simulink model "Model_120S2P"  (R2019b)
settings: Solver=VariableStepAuto  StartTime=0.0  StopTime=800  RelTol=1e-3
libraries: fl_lib x29, nesl_utility x6, simulink x2, hwlogiciolib x1, ee_lib x1
(part 3 of 3)

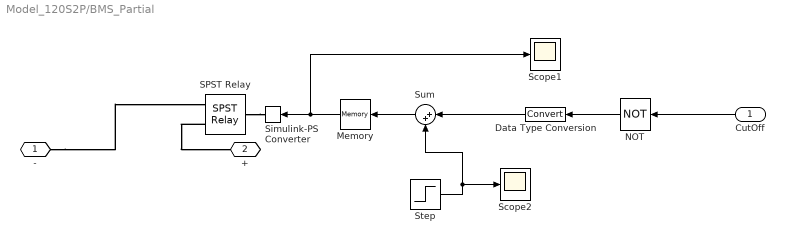
== system Model_120S2P/BMS_Partial ==
  CutOff : Inport
  Data Type Conversion : DataTypeConversion
  Memory : Memory  InheritSampleTime=on  LinearizeMemory=on  LinearizeAsDelay=on
  NOT : Logic  Operator=NOT  IconShape=distinctive  AllPortsSameDT=off  OutDataTypeStr=boolean
  SPST Relay : ee_lib/Switches & Breakers/Relays/SPST Relay  block_choices=ee.enum.controlport.ps  R_closed=0.01 Ohm  G_open=1e-8 1/Ohm  Threshold=0.5  exposemeasurement=ee.enum.exposemeasurement.hidden  T_brk_C_S=0 s  T_mak_C_S=0 s  V_rated=5 V  V_energize=75  V_deenergize=25  l_winding=0.08 H  r_winding=12.5 Ohm  g_winding=1e-9 1/Ohm  enable_faults=ee.enum.relays.enable.no  fault_action=ee.enum.relays.faultaction.none  fault_types=ee.enum.relays.faultTypes.winding  fault_condition_ps=ee.enum.relays.faultConditionSPSTps.csstuck  r_deg_closed_s=1e-9 Ohm  winding_tau_fault=1e-3 s  tau_fault=1e-3 s  enable_temporal_fault=ee.enum.relays.enable.no  t_fault_stick=1 s  t_fault_ComOpen=1 s  t_fault=1 s  enable_behavioral_fault=ee.enum.relays.enable.no  winding_max_permissible_voltage=inf V  n_fail_on_voltage=1  winding_max_permissible_current=inf A  max_permissible_current=inf A  t_fail_on_current=1 s
      settings: SourceProductName=Simscape Electrical  SourceProductBaseCode=PS  InternalSimscapePortConfiguration="{\"Bottom\":[],\"Left\":[{\"id\":\"PS\",\"label\":\"PS\",\"type\":\"input\"}],\"Right\":[{\"id\":\"S\",\"label\":\"S\",\"type\":\"foundation.electrical.electrical\"},{\"id\":\"COM\",\"label\":\"C\",\"type\":\"foundation.electrical.electrical\"}],\"Top\":[]}"
  Scope1 : Scope
  Scope2 : Scope
  Simulink-PS Converter : nesl_utility/Simulink-PS Converter  PhysicalDomain=network_engine_domain  SubClassName=ps_input  LeftPortType=input  RightPortType=output  PseudoPeriodic=off  Frequencies=[]  NoiseDistribution=none  NoiseParameters=[]  Unit=1  AffineConversion=off  FilteringAndDerivatives=provide  SimscapeFilterOrder=1  InputFilterTimeConstant=0.001  UdotUserProvided=0
  Step : Step  Time=10  Before=1  After=0  SampleTime=0
  Sum : Sum  Inputs=|++
  - : PMIOPort  Side=Right
  + : PMIOPort  Port=2  Side=Right
  wires:
  CutOff/1 -> NOT/1
  Memory/1 -> Scope1/1, Simulink-PS Converter/1
  Step/1 -> Scope2/1, Sum/2
  Data Type Conversion/1 -> Sum/1
  NOT/1 -> Data Type Conversion/1
  Sum/1 -> Memory/1
  connections:
  SPST Relay/LConn1 -- Simulink-PS Converter/RConn1
  SPST Relay/RConn2 -- +/RConn1
  -/RConn1 -- SPST Relay/RConn1

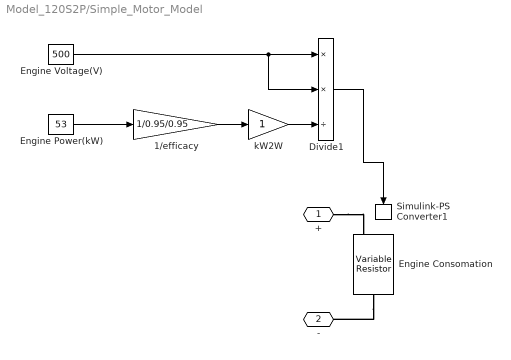
== system Model_120S2P/Simple_Motor_Model ==
  1/efficacy : Gain  Gain=1/0.95/0.95
  Divide1 : Product  Inputs=**/
  Engine Consomation : fl_lib/Electrical/Electrical Elements/Variable Resistor  Rmin=0 Ohm  i_specify=off  i_priority=None  i=0 A  i_nominal_specify=off  i_nominal_unit=A  i_nominal_value=1  v_specify=off  v_priority=None  v=0 V  v_nominal_specify=off  v_nominal_unit=V  v_nominal_value=1
  Engine Power(kW) : Constant  Value=53
  Engine Voltage(V) : Constant  Value=500
  Simulink-PS Converter1 : nesl_utility/Simulink-PS Converter  PhysicalDomain=network_engine_domain  SubClassName=ps_input  LeftPortType=input  RightPortType=output  PseudoPeriodic=off  Frequencies=[]  NoiseDistribution=none  NoiseParameters=[]  Unit=1  AffineConversion=off  FilteringAndDerivatives=provide  SimscapeFilterOrder=1  InputFilterTimeConstant=0.001  UdotUserProvided=0
  kW2W : Gain
  + : PMIOPort  Side=Left
  - : PMIOPort  Port=2  Side=Right
  wires:
  Divide1/1 -> Simulink-PS Converter1/1
  1/efficacy/1 -> kW2W/1
  Engine Voltage(V)/1 -> Divide1/2, Divide1/1
  kW2W/1 -> Divide1/3
  Engine Power(kW)/1 -> 1/efficacy/1
  connections:
  Engine Consomation/RConn1 -- -/RConn1
  +/RConn1 -- Engine Consomation/LConn2
